simulink subsystem "gq_SubSystem"  (R2020b)
settings: Solver=VariableStepAuto  StartTime=0.0  StopTime=10.0  RelTol=1e-3
undefined symbols (not defined in the file): body, g, g1q, mot, Ts
settings Model: Creator=umberto  LastModifiedBy=Musta

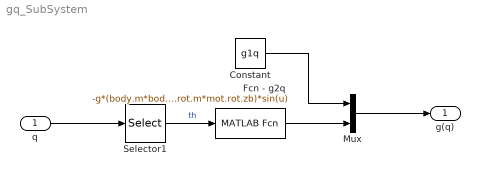
== system gq_SubSystem ==
  q : Inport
  Constant : Constant  Value=g1q  SampleTime=Ts
  Fcn - g2q : MATLABFcn  MATLABFcn=-g*(body.m*body.zb + 2*mot.rot.m*mot.rot.zb)*sin(u)
  Mux : Mux  Inputs=2
  Selector1 : Selector  InputPortWidth=2  IndexOptions=Index vector (dialog)  Indices=[2]  OutputSizes=1
  g(q) : Outport
  wires:
  Selector1/1 -> Fcn - g2q/1  "th"
  q/1 -> Selector1/1
  Constant/1 -> Mux/1
  Mux/1 -> g(q)/1
  Fcn - g2q/1 -> Mux/2
